simulink model "BatteryAgingModel"  (R2018a)
settings: Solver=VariableStepAuto  StartTime=0.0  StopTime=SignalBatt(end,1)  RelTol=0.0017
values from neighbouring files (symbols this model uses):
  Cn = 5.4 * 3600    (= 19440)    [Combined_Optimization.m]    (also in Experimental_BatteryModel.m; Experimental_BatteryModel_Optimized.m; Part45.m)
  DeltaT = 0.1    [Combined_Optimization.m]    (also in Experimental_BatteryModel.m; Experimental_BatteryModel_Optimized.m; Part45.m)
  eta = 1    [Combined_Optimization.m]    (also in Experimental_BatteryModel.m; Experimental_BatteryModel_Optimized.m; Part45.m)
  K0 = param(3)    [Combined_Optimization.m]    (also in Experimental_BatteryModel.m = 3; P3_Skeleton_Graph.m = x(3); Part45.m = 3)
  K1 = param(4)    [Combined_Optimization.m]    (also in Experimental_BatteryModel.m = 0.01; P3_Skeleton_Graph.m = x(4); Part45.m = 0.01)
  K2 = param(5)    [Combined_Optimization.m]    (also in Experimental_BatteryModel.m = 0.01; P3_Skeleton_Graph.m = x(5); Part45.m = 0.01)
  K3 = param(6)    [Combined_Optimization.m]    (also in Experimental_BatteryModel.m = 0.01; P3_Skeleton_Graph.m = x(6); Part45.m = 0.01)
  K4 = param(7)    [Combined_Optimization.m]    (also in Experimental_BatteryModel.m = 0.01; P3_Skeleton_Graph.m = x(7); Part45.m = 0.01)
  R_minusActual = 0.1    [Experimental_BatteryModel.m]    (also in P3_Skeleton_Graph.m = x(2); Part45.m)
  R_plusActual = 0.1    [Experimental_BatteryModel.m]    (also in P3_Skeleton_Graph.m = x(1); Part45.m)
settings Model: Creator=Eduardo  LastModifiedBy=Eduardo

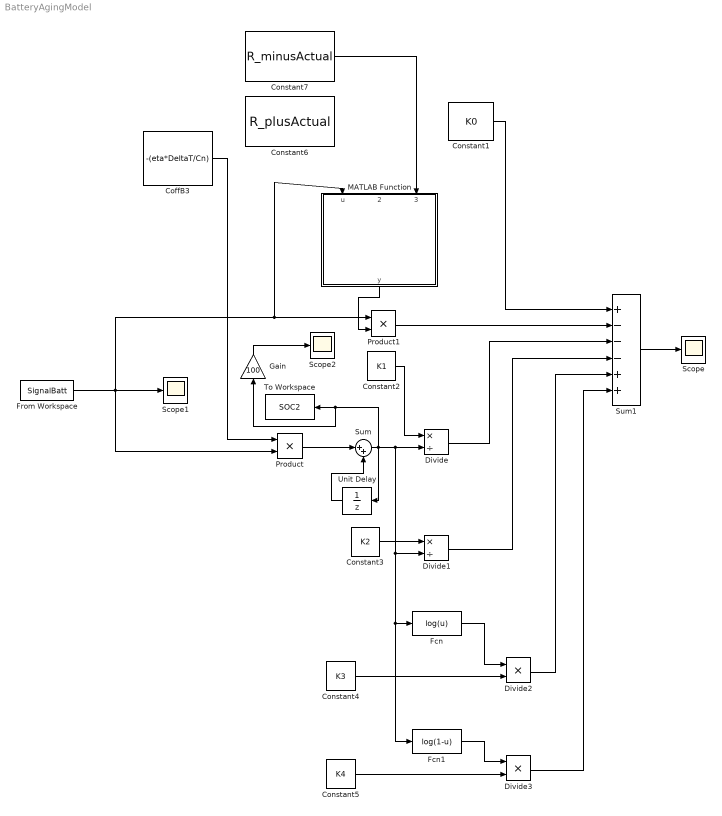
== system BatteryAgingModel ==
  CoffB3 : Constant  Value=-(eta*DeltaT/Cn)
  Constant1 : Constant  Value=K0
  Constant2 : Constant  Value=K1
  Constant3 : Constant  Value=K2
  Constant4 : Constant  Value=K3
  Constant5 : Constant  Value=K4
  Constant6 : Constant  Value=R_plusActual
  Constant7 : Constant  Value=R_minusActual
  Divide : Product  Inputs=*/
  Divide1 : Product  Inputs=*/
  Divide2 : Product  Inputs=**
  Divide3 : Product  Inputs=**
  Fcn : Fcn  Expr=log(u)
  Fcn1 : Fcn  Expr=log(1-u)
  From Workspace : FromWorkspace  VariableName=SignalBatt  OutDataTypeStr=double  SampleTime=0.0001
  Gain : Gain  Gain=100
  MATLAB Function : MATLAB Function  TreatAsAtomicUnit=on
  Product : Product
  Product1 : Product
  Scope : Scope
  Scope1 : Scope
  Scope2 : Scope
  Sum : Sum  Inputs=|++
  Sum1 : Sum  Inputs=+---++
  To Workspace : ToWorkspace  VariableName=SOC2  SaveFormat=Timeseries  SampleTime=-1
  Unit Delay : UnitDelay  InitialCondition=0.9  SampleTime=0.0017
  wires:
  MATLAB Function/1(y) -> Product1/2
  Constant1/1 -> Sum1/1
  Product1/1 -> Sum1/2
  CoffB3/1 -> Product/1
  Product/1 -> Sum/1
  Sum/1 -> Divide1/2, Fcn1/1, Fcn/1, Divide/2, Unit Delay/1, Gain/1, To Workspace/1
  Constant2/1 -> Divide/1
  Divide/1 -> Sum1/3
  Divide1/1 -> Sum1/4
  Constant4/1 -> Divide2/2
  Fcn/1 -> Divide2/1
  Divide2/1 -> Sum1/5
  Fcn1/1 -> Divide3/1
  Constant5/1 -> Divide3/2
  Divide3/1 -> Sum1/6
  Sum1/1 -> Scope/1
  From Workspace/1 -> Product/2, MATLAB Function/1(u), Product1/1, Scope1/1
  Constant7/1 -> MATLAB Function/3(R_minusActual)
  Unit Delay/1 -> Sum/2
  Gain/1 -> Scope2/1
  Constant3/1 -> Divide1/1

== matlab function BatteryAgingModel/MATLAB Function ==
  data: u input; y output; R_plusActual input; R_minusActual input
function y = GetResistance(u, R_plusActual, R_minusActual)
    if u >= 0
        y = R_plusActual;
    else
        y = R_minusActual;
    end
end
